simulink model "es2"  (R2022b)
settings: Solver=VariableStepAuto  StartTime=0.0  StopTime=10.0  RelTol=1e-3
undefined symbols (not defined in the file): A, B, C, D, DiscIntNeverNeededParam, K, Ki, Nu, Nx
settings Model: Creator=david  LastModifiedBy=david

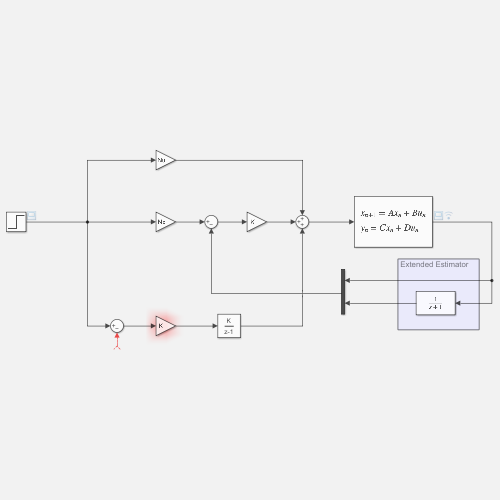
[thumbnail: Simulink's stored preview of the top-level diagram]
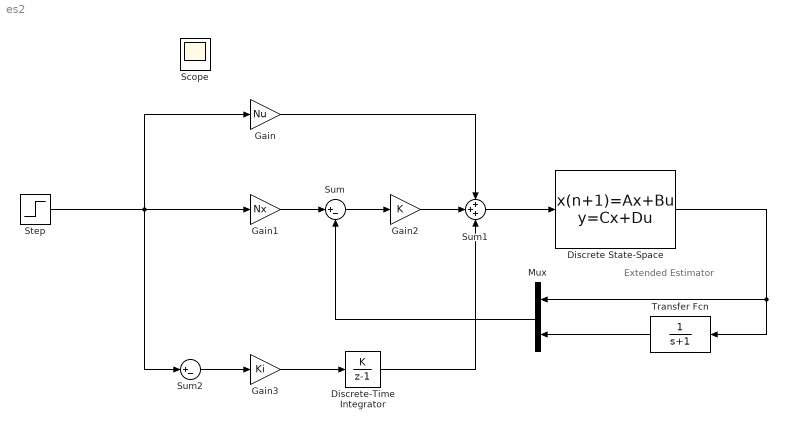
== system es2 ==
  note: Extended Estimator
  Discrete State-Space : DiscreteStateSpace  A=A  B=B  C=C  D=D  SampleTime=-1
  Discrete-Time Integrator : DiscreteIntegrator  IntegratorMethod=Accumulation: Forward Euler  SampleTime=-1  ICPrevOutput=DiscIntNeverNeededParam  ICPrevScaledInput=DiscIntNeverNeededParam
  Gain : Gain  Gain=Nu
  Gain1 : Gain  Gain=Nx
  Gain2 : Gain  Gain=K
  Gain3 : Gain  Gain=Ki
  Mux : Mux  Inputs=2
  Step : Step  SampleTime=0
  Sum : Sum  Inputs=|+-
  Sum1 : Sum  Inputs=+++
  Sum2 : Sum  Inputs=|+-
  Transfer Fcn : TransferFcn  Denominator=[1 1]
  Scope : Scope
  wires:
  Sum/1 -> Gain2/1
  Gain1/1 -> Sum/1
  Gain2/1 -> Sum1/2
  Gain/1 -> Sum1/1
  Sum1/1 -> Discrete State-Space/1
  Gain3/1 -> Discrete-Time Integrator/1
  Discrete-Time Integrator/1 -> Sum1/3
  Step/1 -> Sum2/1, Gain/1, Gain1/1
  Sum2/1 -> Gain3/1
  Discrete State-Space/1 -> Transfer Fcn/1, Mux/1
  Mux/1 -> Sum/2
  Transfer Fcn/1 -> Mux/2
  ? -> Sum2/2
